simulink model "1d ball"  (R2026a)
settings: Solver=VariableStepAuto
settings Model: Creator=tdxt  LastModifiedBy=tdxt

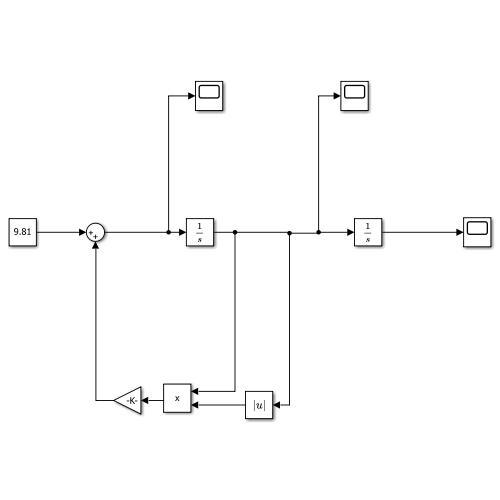
[thumbnail: Simulink's stored preview of the top-level diagram]
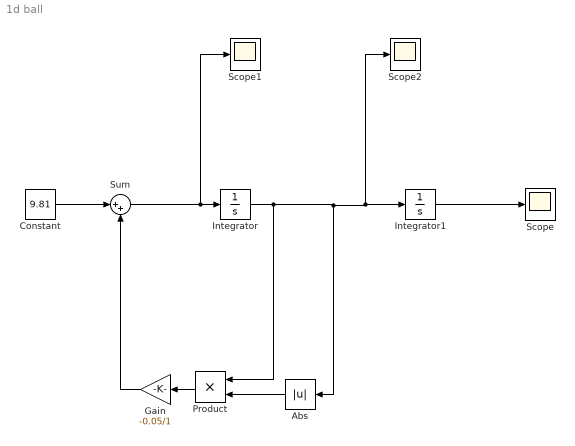
== system 1d ball ==
  Abs : Abs  SaturateOnIntegerOverflow=off
  Constant : Constant  Value=9.81
  Gain : Gain  Gain=-0.05/1
  Integrator : Integrator
  Integrator1 : Integrator
  Product : Product
  Scope : Scope
      settings: ActiveDisplayYMinimum=-15.77606047521115  ActiveDisplayYMaximum=141.98454427690038
  Scope1 : Scope
      settings: ActiveDisplayYMinimum=-1.2262135531352856  ActiveDisplayYMaximum=11.036245950348366
  Scope2 : Scope
      settings: ActiveDisplayYMinimum=-1.7508897383533069  ActiveDisplayYMaximum=15.758007645179767  DataLoggingVariableName=ScopeData2
  Sum : Sum  Inputs=|++
  wires:
  Constant/1 -> Sum/1
  Integrator1/1 -> Scope/1
  Sum/1 -> Scope1/1, Integrator/1
  Integrator/1 -> Product/1, Abs/1, Scope2/1, Integrator1/1
  Gain/1 -> Sum/2
  Abs/1 -> Product/2
  Product/1 -> Gain/1
